simulink subsystem "mission123"  (R2024a)
settings: Solver=VariableStepAuto  StartTime=0.0  StopTime=10.0  RelTol=1e-3
settings Model: Creator=User  LastModifiedBy=User

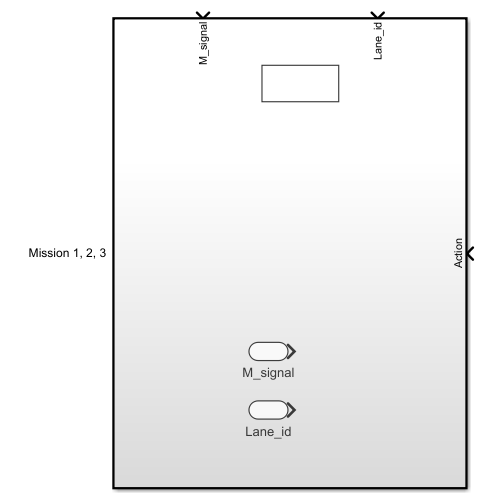
[thumbnail: Simulink's stored preview of the top-level diagram]
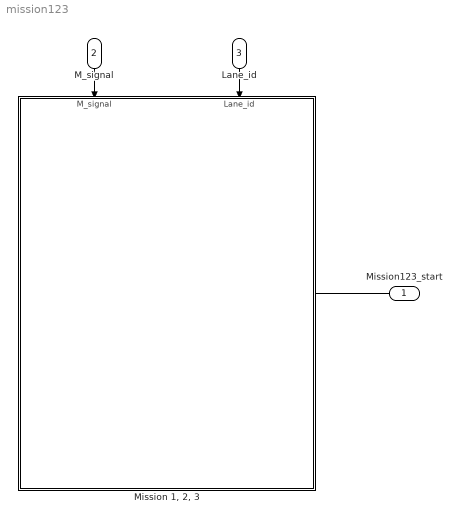
== system mission123 ==
  Mission123_start : Inport
  M_signal : Inport  Port=2
  Lane_id : Inport  Port=3
  "Mission 1, 2, 3" : Subsystem  TreatAsAtomicUnit=on
  wires:
  Mission123_start/1 -> "Mission 1, 2, 3"/Action
  M_signal/1 -> "Mission 1, 2, 3"/1(M_signal)
  Lane_id/1 -> "Mission 1, 2, 3"/2(Lane_id)

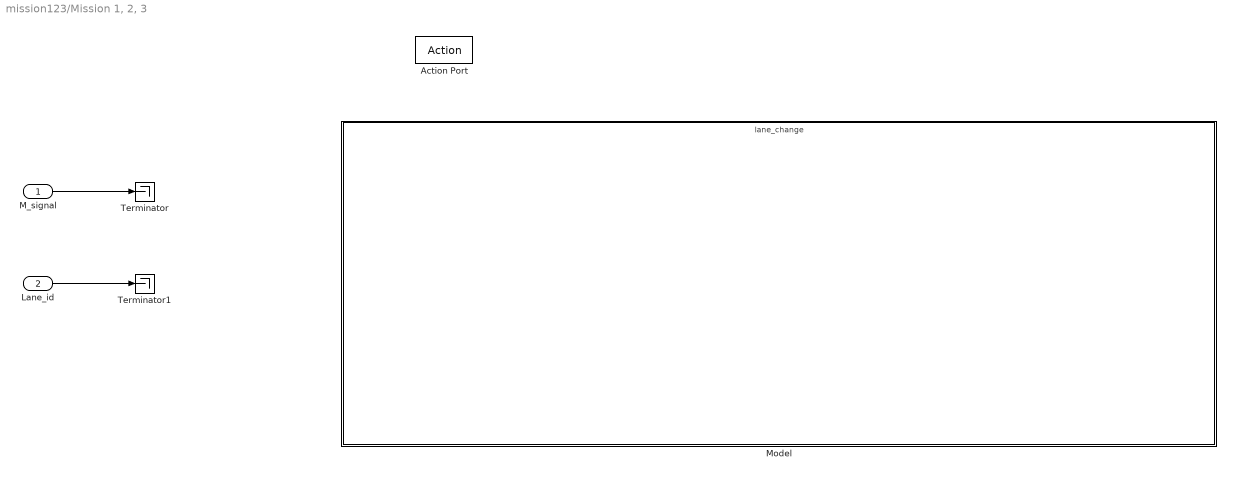
== system mission123/Mission 1, 2, 3 ==
  M_signal : Inport
  Lane_id : Inport  Port=2
  Action Port : ActionPort
  Model : ModelReference  ModelNameDialog=lane_change.slx  SimulationMode=Normal  ModelReferenceVersion=1.5
  Terminator : Terminator
  Terminator1 : Terminator
  wires:
  Lane_id/1 -> Terminator1/1
  M_signal/1 -> Terminator/1
